simulink model "stage2_ddc"  (R2012b)
settings: Solver=FixedStepDiscrete  SolverMode=SingleTasking  StartTime=0.0  StopTime=T  RelTol=1e-3
libraries: xbsIndex_r4 x265, unit_testing x2, r2daq_blocks x1, xps_library x1
settings Model: Creator=ayoung  LastModifiedBy=ayoung
settings DebuggingCC: InheritedTsInSrcMsg=none

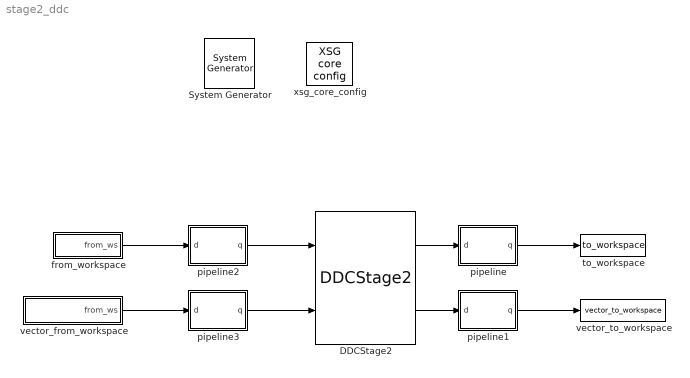
== system stage2_ddc ==
  " System Generator" : xbsIndex_r4/ System Generator  Tag=genX  xilinxfamily=Kintex7  part=xc7k325t  speed=-3  package=fbg676  synthesis_tool=XST  clock_wrapper=Clock Enables  directory=./netlist  proj_type=Project Navigator  Synth_file=XST Defaults  Impl_file=ISE Defaults  testbench=off  simulink_period=1  sysclk_period=10  dcm_input_clock_period=10  incr_netlist=off  trim_vbits=Everywhere in SubSystem  dbl_ovrd=According to Block Masks  core_generation=According to Block Masks  run_coregen=off  deprecated_control=off  eval_field=0  block_type=sysgen
  DDCStage2 : r2daq_blocks/DDCStage2
  from_workspace : Subsystem  AncestorBlock=unit_testing/from_workspace  mask(from_workspace){n_bits=1, bin_pt=0, arith_type=2, var_name=sync_in}
      mask prompts: n_bits "Number of bits"; bin_pt "Binary point"; arith_type "Arithmetic type (ufix=0, fix=1, bool=2)"; var_name "Variable name"
      mask init:
      | blk = from_workspace_init(gcb,...
      |     'n_bits', n_bits,...
      |     'bin_pt',bin_pt,...
      |     'arith_type',arith_type,...
      |     'var_name',var_name);
      mask Display:
      | color('white');
      | text(0.5,0.5,get_param(gcb,'var_name'),'HorizontalAlignment','center');
  pipeline : Subsystem  AncestorBlock=casper_library_delays/pipeline  mask(pipeline){latency=64}
      mask help:
      | An explicitly laid-out delay line to avoid mapping to SRL16s
      | for use in pipelining to help achieve timing closure.
      mask init:
      | pipeline_init(gcb,'latency',latency);
      settings: AttributesFormatString=Latency = %<latency>
      mask Display:
      | port_label('input', 1, 'd');
      | port_label('output', 1, 'q');
      | disp(['Z^-', num2str(latency)]);
  pipeline1 : Subsystem  AncestorBlock=casper_library_delays/pipeline  mask(pipeline){latency=64}
      mask help:
      | An explicitly laid-out delay line to avoid mapping to SRL16s
      | for use in pipelining to help achieve timing closure.
      mask init:
      | pipeline_init(gcb,'latency',latency);
      settings: AttributesFormatString=Latency = %<latency>
      mask Display:
      | port_label('input', 1, 'd');
      | port_label('output', 1, 'q');
      | disp(['Z^-', num2str(latency)]);
  pipeline2 : Subsystem  AncestorBlock=casper_library_delays/pipeline  mask(pipeline){latency=64}
      mask help:
      | An explicitly laid-out delay line to avoid mapping to SRL16s
      | for use in pipelining to help achieve timing closure.
      mask init:
      | pipeline_init(gcb,'latency',latency);
      settings: AttributesFormatString=Latency = %<latency>
      mask Display:
      | port_label('input', 1, 'd');
      | port_label('output', 1, 'q');
      | disp(['Z^-', num2str(latency)]);
  pipeline3 : Subsystem  AncestorBlock=casper_library_delays/pipeline  mask(pipeline){latency=64}
      mask help:
      | An explicitly laid-out delay line to avoid mapping to SRL16s
      | for use in pipelining to help achieve timing closure.
      mask init:
      | pipeline_init(gcb,'latency',latency);
      settings: AttributesFormatString=Latency = %<latency>
      mask Display:
      | port_label('input', 1, 'd');
      | port_label('output', 1, 'q');
      | disp(['Z^-', num2str(latency)]);
  to_workspace : unit_testing/to_workspace  var_name=sync_out
  vector_from_workspace : Subsystem  AncestorBlock=unit_testing/vector_from_workspace  mask(vector_from_workspace){n_in=2, n_bits=25, bin_pt=16, arith_type=1, var_pfx=din_c}
      mask prompts: n_in "Number of inputs"; n_bits "Input width"; bin_pt "Binary point position"; arith_type "Arithmetic type (ufix=0, fix=1, bool=2)"; var_pfx "Variable name prefix"
      mask init:
      | blk = vector_from_workspace_init(gcb,...
      |     'n_in',n_in,...
      |     'n_bits',n_bits,...
      |     'bin_pt',bin_pt,...
      |     'arith_type',arith_type,...
      |     'var_pfx',var_pfx);
      mask Display:
      | color('white');
      | var_pfx = get_param(gcb,'var_pfx');
      | n_1 = 1;
      | n_N = str2num(get_param(gcb,'n_in'));
      | text(0.5,0.5,sprintf('%s_[%d..%d]',var_pfx,n_1,n_N),'HorizontalAlignment','center');
  vector_to_workspace : unit_testing/vector_to_workspace  n_out=2  n_bits=25  bin_pt=16  arith_type=1  var_pfx=dout_c
  xsg_core_config : xps_library/XSG core config  Tag=xps:xsg  hw_sys=ROACH2:sx475t  clk_src=adc0_clk  ROACH_clk_src=sys_clk  ROACH2_clk_src=adc0_clk  MKDIG_clk_src=sys_clk  clk_rate=200  sample_period=1  synthesis_tool=XST
  wires:
  DDCStage2/1 -> pipeline/1(d)
  pipeline/1(q) -> to_workspace/1
  DDCStage2/2 -> pipeline1/1(d)
  pipeline1/1(q) -> vector_to_workspace/1
  from_workspace/1(from_ws) -> pipeline2/1(d)
  pipeline2/1(q) -> DDCStage2/1
  vector_from_workspace/1(from_ws) -> pipeline3/1(d)
  pipeline3/1(q) -> DDCStage2/2

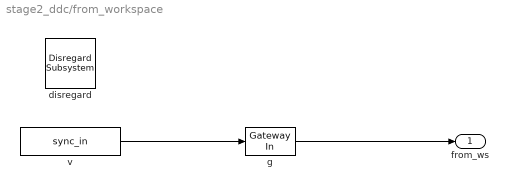
== system stage2_ddc/from_workspace ==
  disregard : xbsIndex_r4/Disregard Subsystem  Tag=discardX  block_type=disregard
  g : xbsIndex_r4/Gateway In  gui_display_data_type=Fixed-point  arith_type=Boolean  n_bits=1  bin_pt=0  preci_type=Single  exp_width=8  frac_width=24  quantization="Round  (unbiased: +/- Inf)"  overflow=Saturate  period=1  dbl_ovrd=off  timing_constraint=None  locs_specified=off  LOCs={}  UseAsADC=off  ADCChannel='1'  inherit_from_input=off  hdl_port=on  block_type=gatewayin
  v : FromWorkspace  VariableName=sync_in  SampleTime=0
  from_ws : Outport
  wires:
  v/1 -> g/1
  g/1 -> from_ws/1

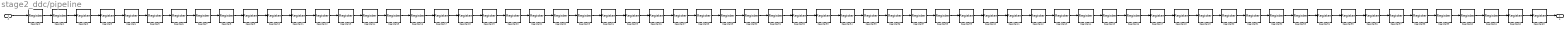
== system stage2_ddc/pipeline ==
  d : Inport
  Register{0..63} (64 alike) : xbsIndex_r4/Register  init=0  rst=off  en=off  dbl_ovrd=off  block_type=register
      Register0 settings: block_version=11.4
      Register1 settings: block_version=11.4
      Register2 settings: block_version=11.4
  q : Outport
  wires:
  Register0/1 -> Register1/1
  Register1/1 -> Register2/1
  Register2/1 -> Register3/1
  Register3/1 -> Register4/1
  Register4/1 -> Register5/1
  Register5/1 -> Register6/1
  Register6/1 -> Register7/1
  Register7/1 -> Register8/1
  Register8/1 -> Register9/1
  Register9/1 -> Register10/1
  Register10/1 -> Register11/1
  Register11/1 -> Register12/1
  Register12/1 -> Register13/1
  Register13/1 -> Register14/1
  Register14/1 -> Register15/1
  Register15/1 -> Register16/1
  Register16/1 -> Register17/1
  Register17/1 -> Register18/1
  Register18/1 -> Register19/1
  Register19/1 -> Register20/1
  Register20/1 -> Register21/1
  Register21/1 -> Register22/1
  Register22/1 -> Register23/1
  Register23/1 -> Register24/1
  Register24/1 -> Register25/1
  Register25/1 -> Register26/1
  Register26/1 -> Register27/1
  Register27/1 -> Register28/1
  Register28/1 -> Register29/1
  Register29/1 -> Register30/1
  Register30/1 -> Register31/1
  Register31/1 -> Register32/1
  Register32/1 -> Register33/1
  Register33/1 -> Register34/1
  Register34/1 -> Register35/1
  Register35/1 -> Register36/1
  Register36/1 -> Register37/1
  Register37/1 -> Register38/1
  Register38/1 -> Register39/1
  Register39/1 -> Register40/1
  Register40/1 -> Register41/1
  Register41/1 -> Register42/1
  Register42/1 -> Register43/1
  Register43/1 -> Register44/1
  Register44/1 -> Register45/1
  Register45/1 -> Register46/1
  Register46/1 -> Register47/1
  Register47/1 -> Register48/1
  Register48/1 -> Register49/1
  Register49/1 -> Register50/1
  Register50/1 -> Register51/1
  Register51/1 -> Register52/1
  Register52/1 -> Register53/1
  Register53/1 -> Register54/1
  Register54/1 -> Register55/1
  Register55/1 -> Register56/1
  Register56/1 -> Register57/1
  Register57/1 -> Register58/1
  Register58/1 -> Register59/1
  Register59/1 -> Register60/1
  Register60/1 -> Register61/1
  Register61/1 -> Register62/1
  Register62/1 -> Register63/1
  d/1 -> Register0/1
  Register63/1 -> q/1

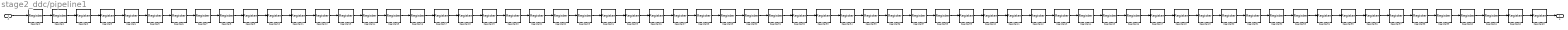
== system stage2_ddc/pipeline1 ==
  d : Inport
  Register{0..63} (64 alike) : xbsIndex_r4/Register  init=0  rst=off  en=off  dbl_ovrd=off  block_type=register
      Register0 settings: block_version=11.4
      Register1 settings: block_version=11.4
      Register2 settings: block_version=11.4
  q : Outport
  wires:
  Register0/1 -> Register1/1
  Register1/1 -> Register2/1
  Register2/1 -> Register3/1
  Register3/1 -> Register4/1
  Register4/1 -> Register5/1
  Register5/1 -> Register6/1
  Register6/1 -> Register7/1
  Register7/1 -> Register8/1
  Register8/1 -> Register9/1
  Register9/1 -> Register10/1
  Register10/1 -> Register11/1
  Register11/1 -> Register12/1
  Register12/1 -> Register13/1
  Register13/1 -> Register14/1
  Register14/1 -> Register15/1
  Register15/1 -> Register16/1
  Register16/1 -> Register17/1
  Register17/1 -> Register18/1
  Register18/1 -> Register19/1
  Register19/1 -> Register20/1
  Register20/1 -> Register21/1
  Register21/1 -> Register22/1
  Register22/1 -> Register23/1
  Register23/1 -> Register24/1
  Register24/1 -> Register25/1
  Register25/1 -> Register26/1
  Register26/1 -> Register27/1
  Register27/1 -> Register28/1
  Register28/1 -> Register29/1
  Register29/1 -> Register30/1
  Register30/1 -> Register31/1
  Register31/1 -> Register32/1
  Register32/1 -> Register33/1
  Register33/1 -> Register34/1
  Register34/1 -> Register35/1
  Register35/1 -> Register36/1
  Register36/1 -> Register37/1
  Register37/1 -> Register38/1
  Register38/1 -> Register39/1
  Register39/1 -> Register40/1
  Register40/1 -> Register41/1
  Register41/1 -> Register42/1
  Register42/1 -> Register43/1
  Register43/1 -> Register44/1
  Register44/1 -> Register45/1
  Register45/1 -> Register46/1
  Register46/1 -> Register47/1
  Register47/1 -> Register48/1
  Register48/1 -> Register49/1
  Register49/1 -> Register50/1
  Register50/1 -> Register51/1
  Register51/1 -> Register52/1
  Register52/1 -> Register53/1
  Register53/1 -> Register54/1
  Register54/1 -> Register55/1
  Register55/1 -> Register56/1
  Register56/1 -> Register57/1
  Register57/1 -> Register58/1
  Register58/1 -> Register59/1
  Register59/1 -> Register60/1
  Register60/1 -> Register61/1
  Register61/1 -> Register62/1
  Register62/1 -> Register63/1
  d/1 -> Register0/1
  Register63/1 -> q/1

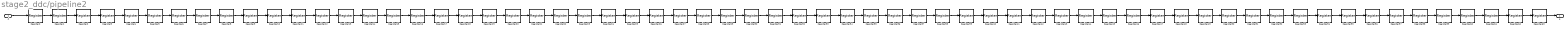
== system stage2_ddc/pipeline2 ==
  d : Inport
  Register{0..63} (64 alike) : xbsIndex_r4/Register  init=0  rst=off  en=off  dbl_ovrd=off  block_type=register
      Register0 settings: block_version=11.4
      Register1 settings: block_version=11.4
      Register2 settings: block_version=11.4
  q : Outport
  wires:
  Register0/1 -> Register1/1
  Register1/1 -> Register2/1
  Register2/1 -> Register3/1
  Register3/1 -> Register4/1
  Register4/1 -> Register5/1
  Register5/1 -> Register6/1
  Register6/1 -> Register7/1
  Register7/1 -> Register8/1
  Register8/1 -> Register9/1
  Register9/1 -> Register10/1
  Register10/1 -> Register11/1
  Register11/1 -> Register12/1
  Register12/1 -> Register13/1
  Register13/1 -> Register14/1
  Register14/1 -> Register15/1
  Register15/1 -> Register16/1
  Register16/1 -> Register17/1
  Register17/1 -> Register18/1
  Register18/1 -> Register19/1
  Register19/1 -> Register20/1
  Register20/1 -> Register21/1
  Register21/1 -> Register22/1
  Register22/1 -> Register23/1
  Register23/1 -> Register24/1
  Register24/1 -> Register25/1
  Register25/1 -> Register26/1
  Register26/1 -> Register27/1
  Register27/1 -> Register28/1
  Register28/1 -> Register29/1
  Register29/1 -> Register30/1
  Register30/1 -> Register31/1
  Register31/1 -> Register32/1
  Register32/1 -> Register33/1
  Register33/1 -> Register34/1
  Register34/1 -> Register35/1
  Register35/1 -> Register36/1
  Register36/1 -> Register37/1
  Register37/1 -> Register38/1
  Register38/1 -> Register39/1
  Register39/1 -> Register40/1
  Register40/1 -> Register41/1
  Register41/1 -> Register42/1
  Register42/1 -> Register43/1
  Register43/1 -> Register44/1
  Register44/1 -> Register45/1
  Register45/1 -> Register46/1
  Register46/1 -> Register47/1
  Register47/1 -> Register48/1
  Register48/1 -> Register49/1
  Register49/1 -> Register50/1
  Register50/1 -> Register51/1
  Register51/1 -> Register52/1
  Register52/1 -> Register53/1
  Register53/1 -> Register54/1
  Register54/1 -> Register55/1
  Register55/1 -> Register56/1
  Register56/1 -> Register57/1
  Register57/1 -> Register58/1
  Register58/1 -> Register59/1
  Register59/1 -> Register60/1
  Register60/1 -> Register61/1
  Register61/1 -> Register62/1
  Register62/1 -> Register63/1
  d/1 -> Register0/1
  Register63/1 -> q/1

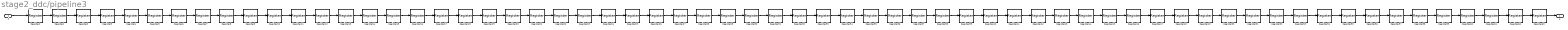
== system stage2_ddc/pipeline3 ==
  d : Inport
  Register{0..63} (64 alike) : xbsIndex_r4/Register  init=0  rst=off  en=off  dbl_ovrd=off  block_type=register
      Register0 settings: block_version=11.4
      Register1 settings: block_version=11.4
      Register2 settings: block_version=11.4
  q : Outport
  wires:
  Register0/1 -> Register1/1
  Register1/1 -> Register2/1
  Register2/1 -> Register3/1
  Register3/1 -> Register4/1
  Register4/1 -> Register5/1
  Register5/1 -> Register6/1
  Register6/1 -> Register7/1
  Register7/1 -> Register8/1
  Register8/1 -> Register9/1
  Register9/1 -> Register10/1
  Register10/1 -> Register11/1
  Register11/1 -> Register12/1
  Register12/1 -> Register13/1
  Register13/1 -> Register14/1
  Register14/1 -> Register15/1
  Register15/1 -> Register16/1
  Register16/1 -> Register17/1
  Register17/1 -> Register18/1
  Register18/1 -> Register19/1
  Register19/1 -> Register20/1
  Register20/1 -> Register21/1
  Register21/1 -> Register22/1
  Register22/1 -> Register23/1
  Register23/1 -> Register24/1
  Register24/1 -> Register25/1
  Register25/1 -> Register26/1
  Register26/1 -> Register27/1
  Register27/1 -> Register28/1
  Register28/1 -> Register29/1
  Register29/1 -> Register30/1
  Register30/1 -> Register31/1
  Register31/1 -> Register32/1
  Register32/1 -> Register33/1
  Register33/1 -> Register34/1
  Register34/1 -> Register35/1
  Register35/1 -> Register36/1
  Register36/1 -> Register37/1
  Register37/1 -> Register38/1
  Register38/1 -> Register39/1
  Register39/1 -> Register40/1
  Register40/1 -> Register41/1
  Register41/1 -> Register42/1
  Register42/1 -> Register43/1
  Register43/1 -> Register44/1
  Register44/1 -> Register45/1
  Register45/1 -> Register46/1
  Register46/1 -> Register47/1
  Register47/1 -> Register48/1
  Register48/1 -> Register49/1
  Register49/1 -> Register50/1
  Register50/1 -> Register51/1
  Register51/1 -> Register52/1
  Register52/1 -> Register53/1
  Register53/1 -> Register54/1
  Register54/1 -> Register55/1
  Register55/1 -> Register56/1
  Register56/1 -> Register57/1
  Register57/1 -> Register58/1
  Register58/1 -> Register59/1
  Register59/1 -> Register60/1
  Register60/1 -> Register61/1
  Register61/1 -> Register62/1
  Register62/1 -> Register63/1
  d/1 -> Register0/1
  Register63/1 -> q/1

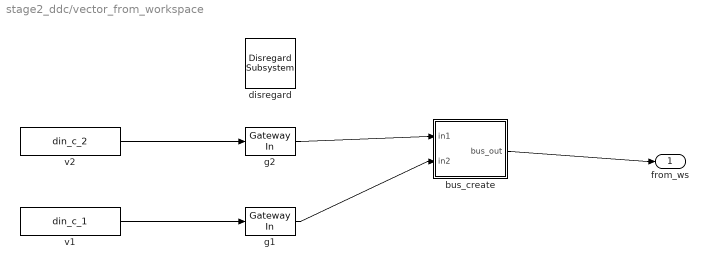
== system stage2_ddc/vector_from_workspace ==
  bus_create : Subsystem  AncestorBlock=casper_library_flow_control/bus_create  mask(bus_create){inputNum=2}
      mask prompts: inputNum "Number of inputs:"
      mask init:
      | bus_create_init(gcb,...
      |     'inputNum', inputNum);
  disregard : xbsIndex_r4/Disregard Subsystem  Tag=discardX  block_type=disregard
  g1 : xbsIndex_r4/Gateway In  gui_display_data_type=Fixed-point  arith_type="Signed  (2's comp)"  n_bits=25  bin_pt=16  preci_type=Single  exp_width=8  frac_width=24  quantization="Round  (unbiased: +/- Inf)"  overflow=Saturate  period=1  dbl_ovrd=off  timing_constraint=None  locs_specified=off  LOCs={}  UseAsADC=off  ADCChannel='1'  inherit_from_input=off  hdl_port=on  block_type=gatewayin
  g2 : xbsIndex_r4/Gateway In  gui_display_data_type=Fixed-point  arith_type="Signed  (2's comp)"  n_bits=25  bin_pt=16  preci_type=Single  exp_width=8  frac_width=24  quantization="Round  (unbiased: +/- Inf)"  overflow=Saturate  period=1  dbl_ovrd=off  timing_constraint=None  locs_specified=off  LOCs={}  UseAsADC=off  ADCChannel='1'  inherit_from_input=off  hdl_port=on  block_type=gatewayin
  v1 : FromWorkspace  VariableName=din_c_1
  v2 : FromWorkspace  VariableName=din_c_2
  from_ws : Outport
  wires:
  v2/1 -> g2/1
  v1/1 -> g1/1
  g2/1 -> bus_create/1(in1)
  g1/1 -> bus_create/2(in2)
  bus_create/1(bus_out) -> from_ws/1

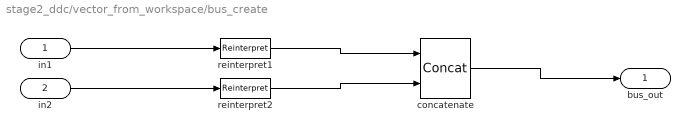
== system stage2_ddc/vector_from_workspace/bus_create ==
  in1 : Inport
  in2 : Inport  Port=2
  concatenate : xbsIndex_r4/Concat  num_inputs=2  dbl_ovrd=off  block_type=concat
  reinterpret1 : xbsIndex_r4/Reinterpret  force_arith_type=on  arith_type=Unsigned  force_bin_pt=on  bin_pt=0  block_type=reinterpret
      settings: infoedit="Changes signal type without altering the binary representation.   You can changed the signal between signed and unsigned, and relocate the binary point.<br><br>Hardware notes: In hardware this block costs nothing.<br><br>Example:  Suppose the input is 6 bits wide, signed, with 2 fractional bits, and the output is forced to unsigned with 0 fractional bits.  Then an input of -2.0 (1110.00 in binary 2's complement) becomes an output of 56 (111000 in binary)."
  reinterpret2 : xbsIndex_r4/Reinterpret  force_arith_type=on  arith_type=Unsigned  force_bin_pt=on  bin_pt=0  block_type=reinterpret
      settings: infoedit="Changes signal type without altering the binary representation.   You can changed the signal between signed and unsigned, and relocate the binary point.<br><br>Hardware notes: In hardware this block costs nothing.<br><br>Example:  Suppose the input is 6 bits wide, signed, with 2 fractional bits, and the output is forced to unsigned with 0 fractional bits.  Then an input of -2.0 (1110.00 in binary 2's complement) becomes an output of 56 (111000 in binary)."
  bus_out : Outport
  wires:
  concatenate/1 -> bus_out/1
  in1/1 -> reinterpret1/1
  reinterpret1/1 -> concatenate/1
  in2/1 -> reinterpret2/1
  reinterpret2/1 -> concatenate/2
